simulink model "error_correct"  (R2020a)
settings: Solver=FixedStepDiscrete  StartTime=0.0  StopTime=20  RelTol=1e-3
settings Model: Creator=shobh  LastModifiedBy=jeeva
settings SolverCC: AutoInsertRateTranBlk=on
settings DataIOCC: LimitDataPoints=on  SaveOutput=off  SignalLogging=off  SaveTime=off
settings OptimizationCC: EnhancedBackFolding=on  PassReuseOutputArgsAs=Individual arguments  ZeroExternalMemoryAtStartup=off  ZeroInternalMemoryAtStartup=off  MaxStackSize=64  OptimizeBlockOrder=speed  DifferentSizesBufferReuse=on  OptimizationCustomize=off  EfficientTunableParamExpr=on
settings DebuggingCC: AlgebraicLoopMsg=error  SingleTaskRateTransMsg=error  ParameterTunabilityLossMsg=error  AllowSymbolicDim=off  SFUnexpectedBacktrackingDiag=warning  SFNoUnconditionalDefaultTransitionDiag=warning  SFExecutionAtInitializationDiag=none  ArithmeticOperatorsInVariantConditions=warning
settings HardwareCC: ProdBitPerPointer=32  ProdBitPerSizeT=32  ProdBitPerPtrDiffT=32  ProdLargestAtomicFloat=None  ProdIntDivRoundTo=Undefined  ProdEndianess=Unspecified  ProdWordSize=32  ProdHWDeviceType=Generic->Unspecified (assume 32-bit Generic)
settings SFSimCC: SimUseLocalCustomCode=off  MATLABDynamicMemAlloc=off  CustomCodeUndefinedFunction=UseInterfaceOnly
settings RTWCC: SystemTargetFile=ert.tlc  HardwareBoard=Robot Operating System (ROS)  TemplateMakefile=ert_default_tmf  RTWUseLocalCustomCode=off  Toolchain=Catkin  TargetLang=C++
settings CodeAppCC: ForceParamTrailComments=on  IgnoreCustomStorageClasses=off  OperatorAnnotations=on  SimulinkDataObjDesc=on  SFDataObjDesc=on  InsertBlockDesc=on
settings ConfigComp: CovMetricSettings=dw  CovHtmlReporting=on  CovSaveCumulativeToWorkspaceVar=on  CovSaveSingleToWorkspaceVar=on  CovExternalEMLEnable=off  CovSFcnEnable=off

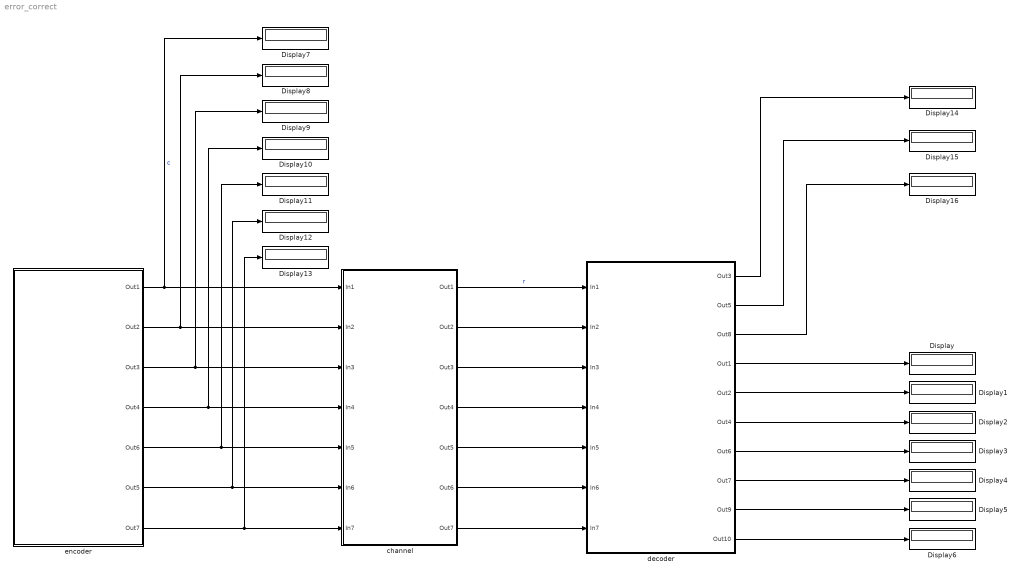
== system error_correct ==
  Display{,1..16} (17 alike) : Display
      settings: Format=binary (Stored Integer)
  channel : Subsystem
  decoder : Subsystem
  encoder : Subsystem
  wires:
  encoder/7(Out7) -> Display13/1, channel/7(In7)
  encoder/2(Out2) -> Display8/1, channel/2(In2)
  encoder/4(Out4) -> Display10/1, channel/4(In4)
  encoder/6(Out5) -> Display12/1, channel/6(In6)
  encoder/1(Out1) -> Display7/1, channel/1(In1)  "c"
  encoder/5(Out6) -> Display11/1, channel/5(In5)
  encoder/3(Out3) -> Display9/1, channel/3(In3)
  decoder/4(Out1) -> Display/1
  decoder/5(Out2) -> Display1/1
  decoder/1(Out3) -> Display14/1
  decoder/6(Out4) -> Display2/1
  decoder/2(Out5) -> Display15/1
  decoder/7(Out6) -> Display3/1
  decoder/8(Out7) -> Display4/1
  decoder/3(Out8) -> Display16/1
  decoder/9(Out9) -> Display5/1
  decoder/10(Out10) -> Display6/1
  channel/1(Out1) -> decoder/1(In1)  "r"
  channel/2(Out2) -> decoder/2(In2)
  channel/3(Out3) -> decoder/3(In3)
  channel/4(Out4) -> decoder/4(In4)
  channel/5(Out5) -> decoder/5(In5)
  channel/6(Out6) -> decoder/6(In6)
  channel/7(Out7) -> decoder/7(In7)

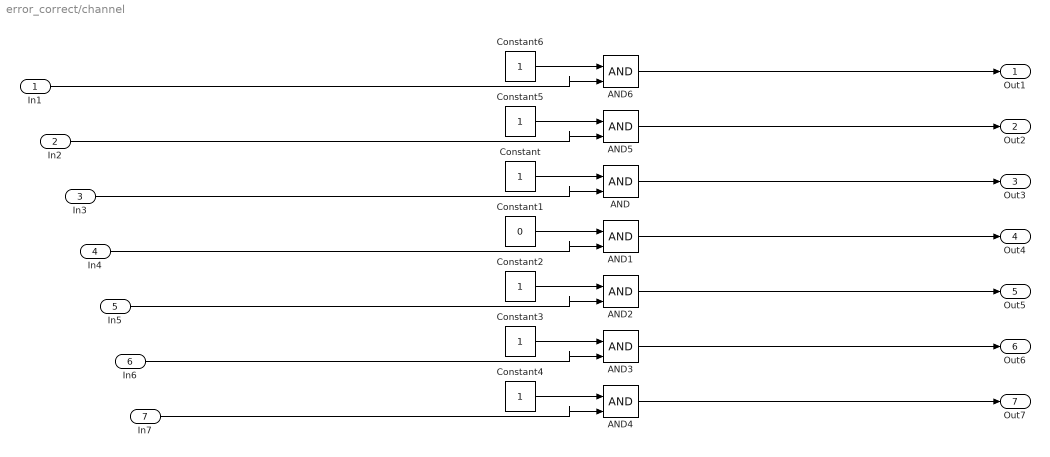
== system error_correct/channel ==
  In1 : Inport
  In2 : Inport  Port=2
  In3 : Inport  Port=3
  In4 : Inport  Port=4
  In5 : Inport  Port=5
  In6 : Inport  Port=6
  In7 : Inport  Port=7
  AND{,1..6} (7 alike) : Logic  IconShape=distinctive  AllPortsSameDT=off  OutDataTypeStr=boolean
  Constant{,2..6} (6 alike) : Constant
  Constant1 : Constant  Value=0
  Out1 : Outport
  Out2 : Outport  Port=2
  Out3 : Outport  Port=3
  Out4 : Outport  Port=4
  Out5 : Outport  Port=5
  Out6 : Outport  Port=6
  Out7 : Outport  Port=7
  wires:
  Constant5/1 -> AND5/1
  AND/1 -> Out3/1
  Constant3/1 -> AND3/1
  Constant/1 -> AND/1
  Constant1/1 -> AND1/1
  AND5/1 -> Out2/1
  Constant2/1 -> AND2/1
  Constant6/1 -> AND6/1
  In1/1 -> AND6/2
  Constant4/1 -> AND4/1
  AND1/1 -> Out4/1
  In6/1 -> AND3/2
  In3/1 -> AND/2
  AND3/1 -> Out6/1
  AND2/1 -> Out5/1
  AND4/1 -> Out7/1
  AND6/1 -> Out1/1
  In2/1 -> AND5/2
  In7/1 -> AND4/2
  In4/1 -> AND1/2
  In5/1 -> AND2/2

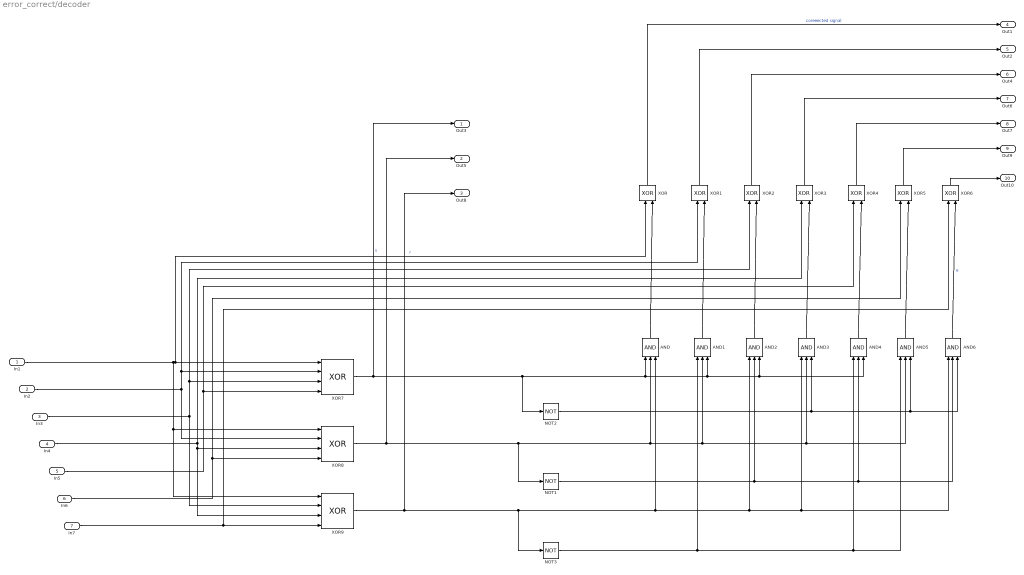
== system error_correct/decoder ==
  In1 : Inport
  In2 : Inport  Port=2
  In3 : Inport  Port=3
  In4 : Inport  Port=4
  In5 : Inport  Port=5
  In6 : Inport  Port=6
  In7 : Inport  Port=7
  AND{,1..6} (7 alike) : Logic  Inputs=3  IconShape=distinctive  AllPortsSameDT=off  OutDataTypeStr=boolean
  NOT1 : Logic  Operator=NOT  IconShape=distinctive  AllPortsSameDT=off  OutDataTypeStr=boolean
  NOT2 : Logic  Operator=NOT  IconShape=distinctive  AllPortsSameDT=off  OutDataTypeStr=boolean
  NOT3 : Logic  Operator=NOT  IconShape=distinctive  AllPortsSameDT=off  OutDataTypeStr=boolean
  XOR{,1..6} (7 alike) : Logic  Operator=XOR  IconShape=distinctive  AllPortsSameDT=off  OutDataTypeStr=boolean
  XOR7 : Logic  Operator=XOR  Inputs=4  IconShape=distinctive  AllPortsSameDT=off  OutDataTypeStr=boolean
  XOR8 : Logic  Operator=XOR  Inputs=4  IconShape=distinctive  AllPortsSameDT=off  OutDataTypeStr=boolean
  XOR9 : Logic  Operator=XOR  Inputs=4  IconShape=distinctive  AllPortsSameDT=off  OutDataTypeStr=boolean
  Out3 : Outport
  Out5 : Outport  Port=2
  Out8 : Outport  Port=3
  Out1 : Outport  Port=4
  Out2 : Outport  Port=5
  Out4 : Outport  Port=6
  Out6 : Outport  Port=7
  Out7 : Outport  Port=8
  Out9 : Outport  Port=9
  Out10 : Outport  Port=10
  wires:
  XOR9/1 -> Out8/1, NOT3/1, AND6/1, AND3/1, AND2/1, AND/3
  NOT2/1 -> AND6/3, AND5/3, AND3/3
  In4/1 -> XOR3/1, XOR9/3, XOR8/3
  In5/1 -> XOR4/1, XOR7/4
  AND2/1 -> XOR2/2
  AND5/1 -> XOR5/2
  In1/1 -> XOR7/1, XOR/1, XOR9/1, XOR8/1  "r"
  XOR8/1 -> Out5/1, NOT1/1, AND5/2, AND3/2, AND1/2, AND/2
  AND1/1 -> XOR1/2
  XOR7/1 -> Out3/1, NOT2/1, AND1/3, AND2/3, AND4/3, AND/1  "s"
  NOT1/1 -> AND6/2, AND4/2, AND2/2
  In3/1 -> XOR9/2, XOR2/1, XOR7/3
  NOT3/1 -> AND1/1, AND4/1, AND5/1
  In6/1 -> XOR5/1, XOR8/4
  XOR5/1 -> Out9/1
  In7/1 -> XOR9/4, XOR6/1
  In2/1 -> XOR8/2, XOR7/2, XOR1/1
  AND4/1 -> XOR4/2
  XOR4/1 -> Out7/1
  AND6/1 -> XOR6/2  "e"
  AND/1 -> XOR/2
  AND3/1 -> XOR3/2
  XOR6/1 -> Out10/1
  XOR1/1 -> Out2/1
  XOR2/1 -> Out4/1
  XOR/1 -> Out1/1  "coreeected signal"
  XOR3/1 -> Out6/1

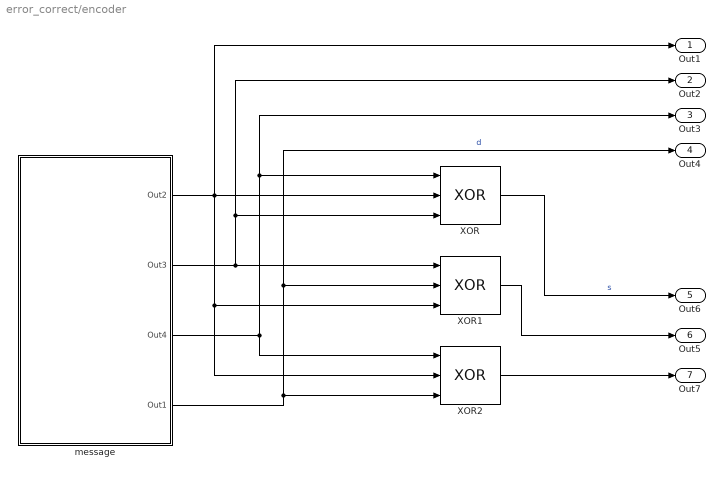
== system error_correct/encoder ==
  XOR : Logic  Operator=XOR  Inputs=3  IconShape=distinctive  AllPortsSameDT=off  OutDataTypeStr=boolean
  XOR1 : Logic  Operator=XOR  Inputs=3  IconShape=distinctive  AllPortsSameDT=off  OutDataTypeStr=boolean
  XOR2 : Logic  Operator=XOR  Inputs=3  IconShape=distinctive  AllPortsSameDT=off  OutDataTypeStr=boolean
  message : Subsystem
  Out1 : Outport
  Out2 : Outport  Port=2
  Out3 : Outport  Port=3
  Out4 : Outport  Port=4
  Out6 : Outport  Port=5
  Out5 : Outport  Port=6
  Out7 : Outport  Port=7
  wires:
  message/1(Out2) -> XOR/2, XOR2/2, XOR1/3, Out1/1
  message/2(Out3) -> XOR1/1, XOR/3, Out2/1
  message/3(Out4) -> XOR2/1, Out3/1, XOR/1
  message/4(Out1) -> XOR1/2, Out4/1, XOR2/3  "d"
  XOR/1 -> Out6/1  "s"
  XOR1/1 -> Out5/1
  XOR2/1 -> Out7/1

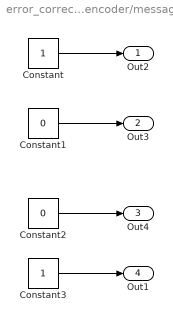
== system error_correct/encoder/message ==
  Constant : Constant
  Constant1 : Constant  Value=0
  Constant2 : Constant  Value=0
  Constant3 : Constant
  Out2 : Outport
  Out3 : Outport  Port=2
  Out4 : Outport  Port=3
  Out1 : Outport  Port=4
  wires:
  Constant/1 -> Out2/1
  Constant1/1 -> Out3/1
  Constant2/1 -> Out4/1
  Constant3/1 -> Out1/1
